simulink model "ur5_controller"  (R2024b)
settings: Solver=ode4  StartTime=0.0  StopTime=20  FixedStep=0.02  MaxStep=0.005  MinStep=0.005  RelTol=1e-3
InitFcn:
  | addpath(genpath(pwd));
libraries: simulink x1
(part 2 of 2)

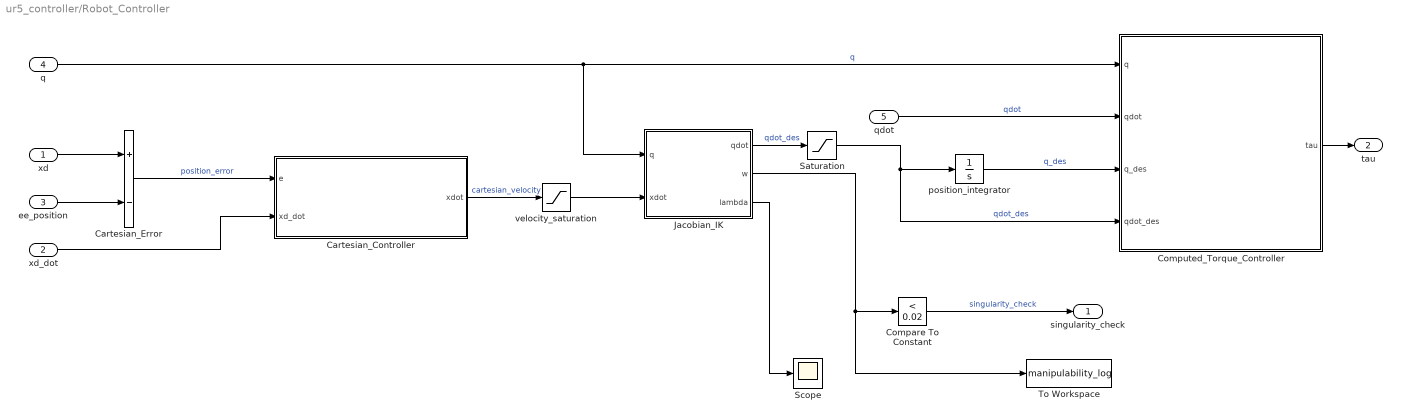
== system ur5_controller/Robot_Controller ==
  xd : Inport
  xd_dot : Inport  Port=2
  ee_position : Inport  Port=3
  q : Inport  Port=4
  qdot : Inport  Port=5
  Cartesian_Controller : MATLAB Function  TreatAsAtomicUnit=on
  Cartesian_Error : Sum  Inputs=+-
  Compare To Constant : simulink/Logic and Bit Operations/Compare To Constant  relop=<  const=0.02  OutDataTypeStr=boolean
  Computed_Torque_Controller : MATLAB Function  TreatAsAtomicUnit=on
  Jacobian_IK : MATLAB Function  TreatAsAtomicUnit=on
  Saturation : Saturate  UpperLimit=2  LowerLimit=-2
  Scope : Scope
  To Workspace : ToWorkspace  VariableName=manipulability_log  SampleTime=-1
  position_integrator : Integrator  InitialCondition=[0; -pi/4; pi/3; -pi/6; pi/4; -pi/2]
  velocity_saturation : Saturate  UpperLimit=0.3  LowerLimit=-0.3
  singularity_check : Outport
  tau : Outport  Port=2
  wires:
  Jacobian_IK/1(qdot) -> Saturation/1  "qdot_des"
  qdot/1 -> Computed_Torque_Controller/2(qdot)  "qdot"
  Cartesian_Controller/1(xdot) -> velocity_saturation/1  "cartesian_velocity"
  q/1 -> Jacobian_IK/1(q), Computed_Torque_Controller/1(q)  "q"
  Cartesian_Error/1 -> Cartesian_Controller/1(e)  "position_error"
  position_integrator/1 -> Computed_Torque_Controller/3(q_des)  "q_des"
  xd/1 -> Cartesian_Error/1
  ee_position/1 -> Cartesian_Error/2
  velocity_saturation/1 -> Jacobian_IK/2(xdot)
  xd_dot/1 -> Cartesian_Controller/2(xd_dot)
  Computed_Torque_Controller/1(tau) -> tau/1
  Saturation/1 -> Computed_Torque_Controller/4(qdot_des), position_integrator/1  "qdot_des"
  Jacobian_IK/2(w) -> To Workspace/1, Compare To Constant/1
  Compare To Constant/1 -> singularity_check/1  "singularity_check"
  Jacobian_IK/3(lambda) -> Scope/1

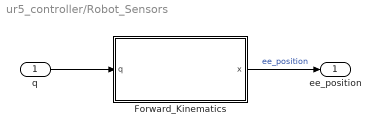
== system ur5_controller/Robot_Sensors ==
  q : Inport
  Forward_Kinematics : MATLAB Function  TreatAsAtomicUnit=on
  ee_position : Outport
  wires:
  Forward_Kinematics/1(x) -> ee_position/1  "ee_position"
  q/1 -> Forward_Kinematics/1(q)

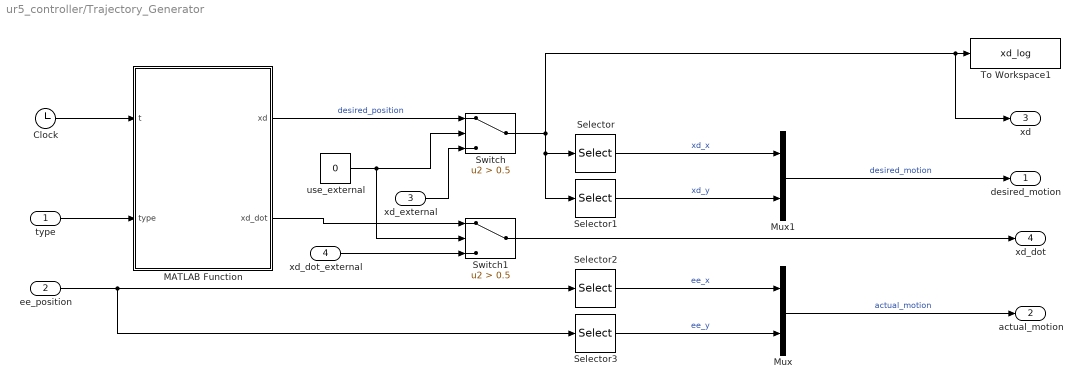
== system ur5_controller/Trajectory_Generator ==
  type : Inport
  ee_position : Inport  Port=2
  xd_external : Inport  Port=3
  xd_dot_external : Inport  Port=4
  Clock : Clock
  MATLAB Function : MATLAB Function  TreatAsAtomicUnit=on
  Mux : Mux  Inputs=2
  Mux1 : Mux  Inputs=2
  Selector : Selector  InputPortWidth=3  IndexOptions=Index vector (dialog)  Indices=[1]  OutputSizes=1
  Selector1 : Selector  InputPortWidth=3  IndexOptions=Index vector (dialog)  Indices=[2]  OutputSizes=1
  Selector2 : Selector  InputPortWidth=3  IndexOptions=Index vector (dialog)  Indices=[1]  OutputSizes=1
  Selector3 : Selector  InputPortWidth=3  IndexOptions=Index vector (dialog)  Indices=[2]  OutputSizes=1
  Switch : Switch  Criteria=u2 > Threshold  Threshold=0.5  SaturateOnIntegerOverflow=off  InputSameDT=off
  Switch1 : Switch  Criteria=u2 > Threshold  Threshold=0.5  SaturateOnIntegerOverflow=off  InputSameDT=off
  To Workspace1 : ToWorkspace  VariableName=xd_log  SampleTime=-1
  use_external : Constant  Value=0
  desired_motion : Outport
  actual_motion : Outport  Port=2
  xd : Outport  Port=3
  xd_dot : Outport  Port=4
  wires:
  Selector2/1 -> Mux/1  "ee_x"
  Selector3/1 -> Mux/2  "ee_y"
  Selector1/1 -> Mux1/2  "xd_y"
  Clock/1 -> MATLAB Function/1(t)
  Selector/1 -> Mux1/1  "xd_x"
  ee_position/1 -> Selector3/1, Selector2/1
  Mux1/1 -> desired_motion/1  "desired_motion"
  Mux/1 -> actual_motion/1  "actual_motion"
  type/1 -> MATLAB Function/2(type)
  use_external/1 -> Switch/2, Switch1/2
  xd_external/1 -> Switch/3
  MATLAB Function/1(xd) -> Switch/1  "desired_position"
  Switch/1 -> xd/1, To Workspace1/1, Selector/1, Selector1/1
  xd_dot_external/1 -> Switch1/3
  MATLAB Function/2(xd_dot) -> Switch1/1
  Switch1/1 -> xd_dot/1

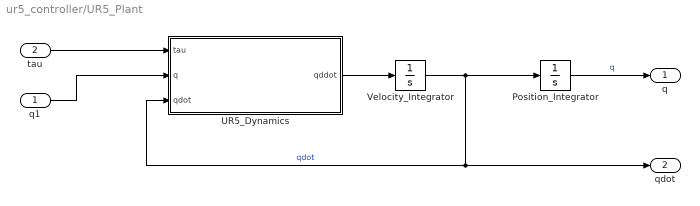
== system ur5_controller/UR5_Plant ==
  q1 : Inport
  tau : Inport  Port=2
  Position_Integrator : Integrator  InitialCondition=[0; -pi/4; pi/3; -pi/6; pi/4; -pi/2]
  UR5_Dynamics : MATLAB Function  TreatAsAtomicUnit=on
  Velocity_Integrator : Integrator  InitialCondition=zeros(6,1)
  q : Outport
  qdot : Outport  Port=2
  wires:
  tau/1 -> UR5_Dynamics/1(tau)
  q1/1 -> UR5_Dynamics/2(q)
  UR5_Dynamics/1(qddot) -> Velocity_Integrator/1
  Velocity_Integrator/1 -> qdot/1, UR5_Dynamics/3(qdot), Position_Integrator/1  "qdot"
  Position_Integrator/1 -> q/1  "q"

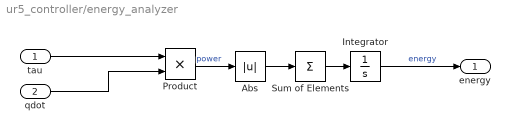
== system ur5_controller/energy_analyzer ==
  tau : Inport
  qdot : Inport  Port=2
  Abs : Abs  SaturateOnIntegerOverflow=off
  Integrator : Integrator
  Product : Product
  Sum of Elements : Sum  Inputs=+
  energy : Outport
  wires:
  Sum of Elements/1 -> Integrator/1
  Abs/1 -> Sum of Elements/1
  qdot/1 -> Product/2
  Product/1 -> Abs/1  "power"
  tau/1 -> Product/1
  Integrator/1 -> energy/1  "energy"

== matlab function ur5_controller/Robot_Controller/Jacobian_IK ==
  data: q input; qdot output; xdot input; w output; lambda output
function [qdot, w, lambda] = Jacobian_IK(q, xdot)

J = jacobian_ur5(q');

% manipulability using singular values
s = svd(J);
w = prod(s);

lambda_min = 0.001;
lambda_max = 0.05;
k = 0.002;
epsilon = 1e-6;

lambda = lambda_min + k/(w + epsilon);
lambda = min(lambda, lambda_max);

v = [xdot; zeros(3,1)];
qdot = J' * ((J*J' + lambda^2 * eye(6)) \ v);

end

== matlab function ur5_controller/Robot_Controller/Cartesian_Controller ==
  data: e input; xdot output; xd_dot input
function xdot = Cartesian_Controller(e, xd_dot)

Kp = 3;

xdot = xd_dot + Kp*e;

end

== matlab function ur5_controller/Robot_Sensors/Forward_Kinematics ==
  data: q input; x output
function x = Forward_Kinematics(q)

% Force output size
x = zeros(3,1);

[~,~,~,~,~,T] = forward_chain_ur5(q');

x = T(1:3,4);

end

== matlab function ur5_controller/UR5_Plant/UR5_Dynamics ==
  data: tau input; qddot output; q input; qdot input
function qddot = UR5_Dynamics(tau,q,qdot)

qddot = zeros(6,1);

M = mass_matrix_ur5(q');
C = coriolis_ur5(q',qdot');
G = gravity_ur5(q');

qddot = M \ (tau - C*qdot - G);

end

== matlab function ur5_controller/Robot_Controller/Computed_Torque_Controller ==
  data: q input; tau output; qdot input; q_des input; qdot_des input
function tau  = Computed_Torque_Controller(q,qdot,q_des,qdot_des)

Kp = 50*eye(6);
Kd = 10*eye(6);

e  = q_des - q;
ed = qdot_des - qdot;

qdd_cmd = Kp*e + Kd*ed;

M = mass_matrix_ur5(q');
C = coriolis_ur5(q',qdot');
G = gravity_ur5(q');

tau_m = M*qdd_cmd;
tau_c = C*qdot;
tau_g = G;

tau = tau_m + tau_c + tau_g;

end

== matlab function ur5_controller/Trajectory_Generator/MATLAB Function ==
  data: xd output; t input; xd_dot output; type input
function [xd, xd_dot] = Trajectory_Generator(t, type)

% Pre-initialize outputs (VERY IMPORTANT for Simulink)
xd = zeros(3,1);
xd_dot = zeros(3,1);

% trajectory parameters
r = 0.1;
cx = 0.3;
cy = 0.2;
z = 0.4;
w = 0.5;

switch type

    case 1 % Circle

        x = cx + r*cos(w*t);
        y = cy + r*sin(w*t);

        xd = [x;y;z];

        xd_dot = [-r*w*sin(w*t);
                   r*w*cos(w*t);
                   0];

    case 2 % Square

    a = r;
    k = 5;
    
    x = cx + a * tanh(k*cos(w*t));
    y = cy + a * tanh(k*sin(w*t));
    
    xd = [x;y;z];
    
    xd_dot = [
    -a*k*w*sin(w*t)*(1-tanh(k*cos(w*t))^2)
     a*k*w*cos(w*t)*(1-tanh(k*sin(w*t))^2)
     0];

    case 3 % Figure-8

        x = cx + r*sin(w*t);
        y = cy + r*sin(w*t)*cos(w*t);

        xd = [x;y;z];

        xd_dot = [r*w*cos(w*t);
                  r*w*cos(2*w*t);
                  0];

    case 4 % Upward Spiral

    r_spiral = 0.02*t;
    
    x = cx + r_spiral*cos(w*t);
    y = cy + r_spiral*sin(w*t);
    z = 0.4 + 0.02*t;
    
    xd = [x;y;z];
    
    xd_dot = [
    -r_spiral*w*sin(w*t) + 0.02*cos(w*t)
     r_spiral*w*cos(w*t) + 0.02*sin(w*t)
     0.02];

end

end
